simulink model "ISS"  (R2018a)
settings: Solver=FixedStepAuto  StartTime=0.0  StopTime=1*24*3600  FixedStep=10  RelTol=1e-3
values from neighbouring files (symbols this model uses):
  a = -mu/(2*xi)    [AA279A_ECI2OE.m]    (also in AA279A_HW2.m = rp/(1-e(ii)); ECI2OE.m = inf; Halleys_Comet_Call.m = 2667966400; ISS_Call.m = 6781.5)
  e = norm(e_vec)    [AA279A_ECI2OE.m]    (also in AA279A_HW2.m = [0.7 0.0 1.9 1.0]; ECI2OE.m = norm(eVec); Halleys_Comet_Call.m = 0.967; ISS_Call.m = 0.0006483)
  i = acosd(h(3)/hnorm)    [AA279A_ECI2OE.m]    (also in ECI2OE.m = acosd(hVec(3)/h); ISS_Call.m = 0.901326422973; Iridium18_Call.m = 1.50785975397; Molniya331_Call.m = deg2rad(i))
  InitialDate = [2018, 4, 22]    [ISS_Call.m]    (also in Iridium18_Call.m = 57421.510593; Molniya331_Call.m = [2018, 2, 1])
  M0 = 0    [Halleys_Comet_Call.m]    (also in ISS_Call.m = 0.9101; Iridium18_Call.m = 0.475253155318; Molniya331_Call.m = E - e*sin(E))
  n = [-h(2);h(1);0]    [AA279A_ECI2OE.m]    (also in AA279A_OE2ECI.m = sqrt(mu/a^3); ECI2OE.m = norm(nVec); Halleys_Comet_Call.m = sqrt(mu/(a^3)); ISS_Call.m = sqrt(mu/(a^3)))
  RAAN = RAAN + 360    [AA279A_ECI2OE.m]    (also in ISS_Call.m = 1.41506932429; Iridium18_Call.m = 4.02952891054; Molniya331_Call.m = deg2rad(RAAN))
  w = 360 - w    [AA279A_ECI2OE.m]    (also in ECI2OE.m; ISS_Call.m = 0.685300040137; Iridium18_Call.m = 1.56927789035; Molniya331_Call.m = deg2rad(w))
settings Model: Creator=Marquito  LastModifiedBy=Marquito

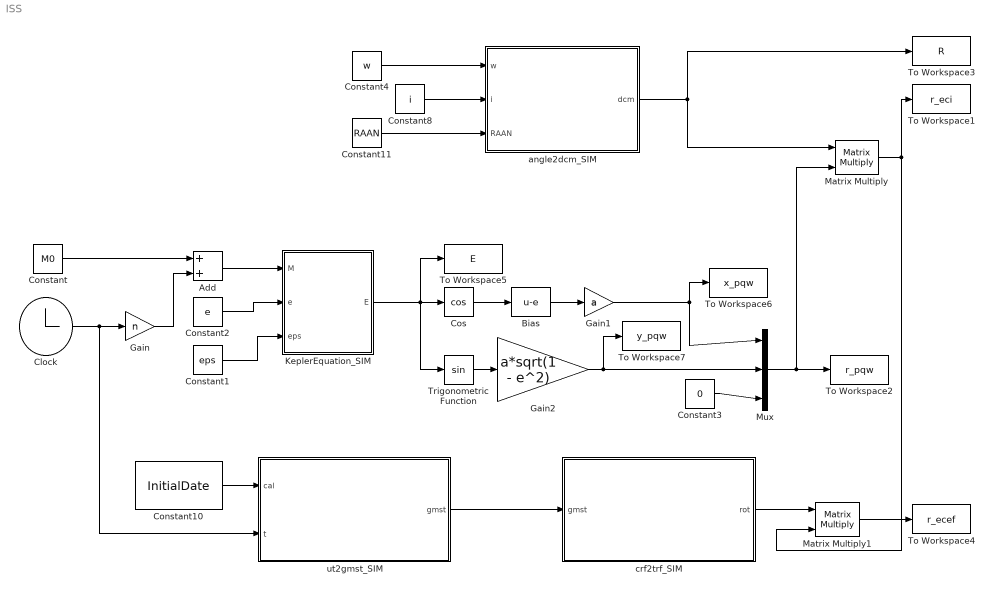
== system ISS ==
  Add : Sum
  Bias : Bias  Bias=-e
  Clock : Clock
  Constant : Constant  Value=M0
  Constant1 : Constant  Value=eps
  Constant10 : Constant  Value=InitialDate
  Constant11 : Constant  Value=RAAN
  Constant2 : Constant  Value=e
  Constant3 : Constant  Value=0
  Constant4 : Constant  Value=w
  Constant8 : Constant  Value=i
  Cos : Trigonometry  Operator=cos
  Gain : Gain  Gain=n
  Gain1 : Gain  Gain=a
  Gain2 : Gain  Gain=a*sqrt(1 - e^2)
  KeplerEquation_SIM : MATLAB Function  TreatAsAtomicUnit=on
  Matrix Multiply : Product  Multiplication=Matrix(*)
  Matrix Multiply1 : Product  Multiplication=Matrix(*)
  Mux : Mux  Inputs=3
  To Workspace1 : ToWorkspace  VariableName=r_eci  SampleTime=-1
  To Workspace2 : ToWorkspace  VariableName=r_pqw  SampleTime=-1
  To Workspace3 : ToWorkspace  VariableName=R  SampleTime=-1
  To Workspace4 : ToWorkspace  VariableName=r_ecef  SampleTime=-1
  To Workspace5 : ToWorkspace  VariableName=E  SampleTime=-1
  To Workspace6 : ToWorkspace  VariableName=x_pqw  SampleTime=-1
  To Workspace7 : ToWorkspace  VariableName=y_pqw  SampleTime=-1
  Trigonometric Function : Trigonometry
  angle2dcm_SIM : MATLAB Function  TreatAsAtomicUnit=on
  crf2trf_SIM : MATLAB Function  TreatAsAtomicUnit=on
  ut2gmst_SIM : MATLAB Function  TreatAsAtomicUnit=on
  wires:
  Clock/1 -> Gain/1, ut2gmst_SIM/2(t)
  Add/1 -> KeplerEquation_SIM/1(M)
  KeplerEquation_SIM/1(E) -> Trigonometric Function/1, To Workspace5/1, Cos/1
  Constant2/1 -> KeplerEquation_SIM/2(e)
  Constant1/1 -> KeplerEquation_SIM/3(eps)
  angle2dcm_SIM/1(dcm) -> To Workspace3/1, Matrix Multiply/1
  Constant10/1 -> ut2gmst_SIM/1(cal)
  ut2gmst_SIM/1(gmst) -> crf2trf_SIM/1(gmst)
  crf2trf_SIM/1(rot) -> Matrix Multiply1/1
  Matrix Multiply1/1 -> To Workspace4/1
  Constant/1 -> Add/1
  Gain/1 -> Add/2
  Cos/1 -> Bias/1
  Bias/1 -> Gain1/1
  Gain1/1 -> To Workspace6/1, Mux/1
  Trigonometric Function/1 -> Gain2/1
  Gain2/1 -> To Workspace7/1, Mux/2
  Constant3/1 -> Mux/3
  Mux/1 -> To Workspace2/1, Matrix Multiply/2
  Matrix Multiply/1 -> Matrix Multiply1/2, To Workspace1/1
  Constant8/1 -> angle2dcm_SIM/2(i)
  Constant11/1 -> angle2dcm_SIM/3(RAAN)
  Constant4/1 -> angle2dcm_SIM/1(w)

== matlab function ISS/KeplerEquation_SIM ==
  data: M input; E output; e input; eps input
function E = KeplerEq(M,e,eps)
% Function solves Kepler's equation M = E-e*sin(E)
% Input - Mean Anomaly M [rad], Eccentricity e, and Epsilon 
% Output - Eccentric anomaly E [rad] 

En  = M;
Ens = En - (En-e*sin(En)- M)/(1 - e*cos(En));
while ( abs(Ens-En) > eps )
	En = Ens;
	Ens = En - (En - e*sin(En) - M)/(1 - e*cos(En));
end
E = Ens;
end

== matlab function ISS/ut2gmst_SIM ==
  data: cal input; t input; gmst output
function gmst = ut2gmst(cal, t)
% ut2gmst  Converts  from  UT1  time to GMST
%
% Inputs:
%     cal - vector  containing  simulation  start  date as [YYYY , MM, DD]
%            Note: the  day  should  be a decimal  value  accounting for  
%            the  start time of the  simulation
%       t - current  time in  seconds (from  Simulink  clock  source)
%
% Outputs:
%    gmst - current  Greenwich  Mean  Sidereal  Time [rad]

year = cal(1);
month = cal(2);
startDay = cal(3);

day = startDay + t/86400;
mjd = cal2mjd(month, day, year);
gmst = mjd2gmst(mjd);

end

== matlab function ISS/angle2dcm_SIM ==
  data: w input; i input; dcm output; RAAN input
function dcm  = angle2dcm(w, i, RAAN)
% dcm = angle2dcm(r1,r2,r3,seq)
% builds euler angle rotation matrix
% 
% r = [r1 r2 r3]
% seq = 'ZYX' (default)
%       'ZXZ'
% dcm = direction cosine matrix

dcm = eye(3,3);
r = [-w; -i; -RAAN];
seq = 'ZXZ';

switch seq
  case 'ZYX'
    dcm = Tx(r(3))*Ty(r(2))*Tz(r(1));
  case 'ZXZ'
    dcm = Tz(r(3))*Tx(r(2))*Tz(r(1)); 
end

function A = Tx(a)
A = [1 0 0;
    0 cos(a) sin(a);
    0 -sin(a) cos(a)];
end

function A = Ty(a)
A = [cos(a) 0 -sin(a);
    0 1 0;
    sin(a) 0 cos(a)];
end

function A = Tz(a)
A = [cos(a) sin(a) 0;
    -sin(a) cos(a) 0;
    0 0 1];
end

end

== matlab function ISS/crf2trf_SIM ==
  data: gmst input; rot output
function rot = crf2trf(gmst)
% crf2trf  Creates a rotation  matrix  between  CRF  and  TRFsystems
%
% Inputs:
%    gmst - Greenwich  Mean  Sidereal  Time [rad]
%
% Outputs:
%    rot   - rotation  matrix  from  celestial  to  terrestrial reference  
%            frames

rot = rotz(-gmst);

end
